simulink model "hexa_control"  (R2021a)
settings: Solver=VariableStepAuto  StartTime=0.0  StopTime=inf  RelTol=1e-3
StartFcn:
  | mikro.start('-a');
StopFcn:
  | mikro.stop();
values from neighbouring files (symbols this model uses):
  basic_time_step = 0.005    [Initialization.m]
  F = [F1; F2]    [Initialization.m]
  g = 9.81    [Initialization.m]
  J = diag([82973.961,81490.708,157588.499]*10^(-6))    [Initialization.m]
  K_p = K_p_scalar*eye(3)    [Initialization.m]
  K_R = K_R_scalar*eye(3)    [Initialization.m]
  K_v = K_v_scalar*eye(3)    [Initialization.m]
  K_w = K_w_scalar*eye(3)    [Initialization.m]
  m = 0.395 + 1.870    (= 2.265)    [Initialization.m]
  motion_capture_rate = 0.01    [Initialization.m]
undefined symbols (not defined in the file or in its folder): DiscIntNeverNeededParam, init
libraries: genomix x5, simulink x4, sharedTrackingLibrary x1
PauseFcn:
  | mikro.stop();
settings Model: Creator=nicola  LastModifiedBy=nicola

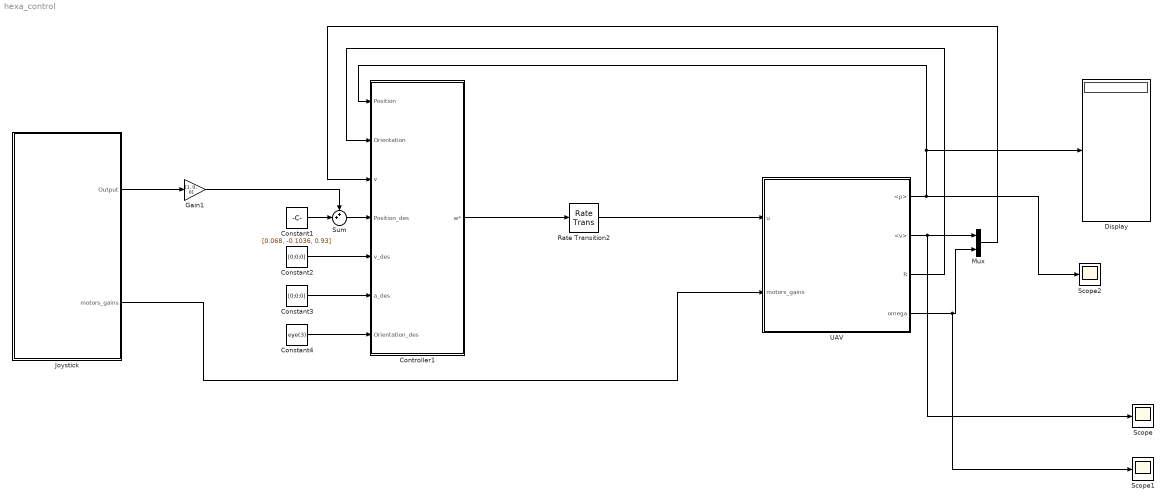
== system hexa_control ==
  Constant1 : Constant  Value=[0.068, -0.1036, 0.93]
  Constant2 : Constant  Value=[0;0;0]
  Constant3 : Constant  Value=[0;0;0]
  Constant4 : Constant  Value=eye(3)
  Controller1 : Subsystem
  Display : Display
  Gain1 : Gain  Gain=[1, 0, 0]
  Joystick : Subsystem
  Mux : Mux  Inputs=2
  Rate Transition2 : RateTransition  Integrity=off
  Scope : Scope
  Scope1 : Scope
  Scope2 : Scope
  Sum : Sum  Inputs=++|
  UAV : Subsystem
  wires:
  Controller1/1("w* ") -> Rate Transition2/1
  Constant3/1 -> Controller1/6(a_des)
  Constant1/1 -> Sum/2
  Gain1/1 -> Sum/1
  Constant2/1 -> Controller1/5(v_des)
  Sum/1 -> Controller1/4(Position_des)
  UAV/1(<p>) -> Scope2/1, Display/1, Controller1/1(Position)
  Constant4/1 -> Controller1/7(Orientation_des)
  UAV/3(R) -> Controller1/2(Orientation)
  Rate Transition2/1 -> UAV/1(u)
  UAV/2(<v>) -> Scope/1, Mux/1
  UAV/4(omega) -> Scope1/1, Mux/2
  Mux/1 -> Controller1/3(v)
  Joystick/1(Output) -> Gain1/1
  Joystick/2(motors_gains) -> UAV/2(motors_gains)

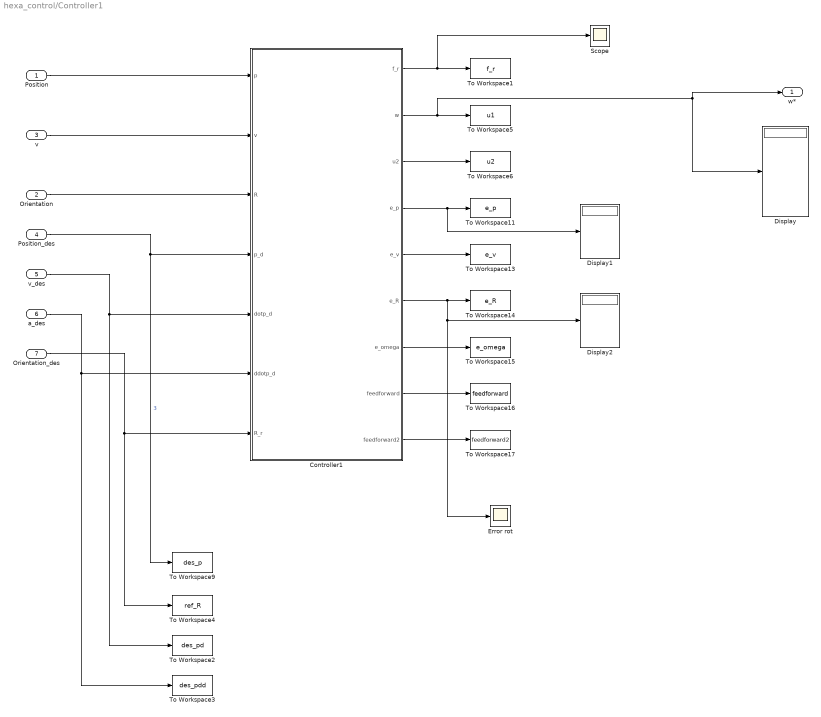
== system hexa_control/Controller1 ==
  Position : Inport
  Orientation : Inport  Port=2
  v : Inport  Port=3
  Position_des : Inport  Port=4
  v_des : Inport  Port=5
  a_des : Inport  Port=6
  Orientation_des : Inport  Port=7
  Controller1 : MATLAB Function  TreatAsAtomicUnit=on
  Display : Display
  Display1 : Display
  Display2 : Display
  Error rot : Scope
  Scope : Scope
  To Workspace1 : ToWorkspace  VariableName=f_r  SaveFormat=Timeseries  SampleTime=-1
  To Workspace11 : ToWorkspace  VariableName=e_p  SaveFormat=Timeseries  SampleTime=-1
  To Workspace13 : ToWorkspace  VariableName=e_v  SaveFormat=Timeseries  SampleTime=-1
  To Workspace14 : ToWorkspace  VariableName=e_R  SaveFormat=Timeseries  SampleTime=-1
  To Workspace15 : ToWorkspace  VariableName=e_omega  SaveFormat=Timeseries  SampleTime=-1
  To Workspace16 : ToWorkspace  VariableName=feedforward  SaveFormat=Timeseries  SampleTime=-1
  To Workspace17 : ToWorkspace  VariableName=feedforward2  SaveFormat=Timeseries  SampleTime=-1
  To Workspace2 : ToWorkspace  VariableName=des_pd  SaveFormat=Timeseries  SampleTime=-1
  To Workspace3 : ToWorkspace  VariableName=des_pdd  SaveFormat=Timeseries  SampleTime=-1
  To Workspace4 : ToWorkspace  VariableName=ref_R  SaveFormat=Timeseries  SampleTime=-1
  To Workspace5 : ToWorkspace  VariableName=u1  SaveFormat=Timeseries  SampleTime=-1
  To Workspace6 : ToWorkspace  VariableName=u2  SaveFormat=Timeseries  SampleTime=-1
  To Workspace9 : ToWorkspace  VariableName=des_p  SaveFormat=Timeseries  SampleTime=-1
  "w* " : Outport
  wires:
  Position/1 -> Controller1/1(p)
  v/1 -> Controller1/2(v)
  Orientation_des/1 -> To Workspace4/1, Controller1/7(R_r)
  Orientation/1 -> Controller1/3(R)
  Position_des/1 -> Controller1/4(p_d), To Workspace9/1  "3"
  v_des/1 -> Controller1/5(dotp_d), To Workspace2/1
  a_des/1 -> Controller1/6(ddotp_d), To Workspace3/1
  Controller1/4(e_p) -> Display1/1, To Workspace11/1
  Controller1/5(e_v) -> To Workspace13/1
  Controller1/7(e_omega) -> To Workspace15/1
  Controller1/3(u2) -> To Workspace6/1
  Controller1/2(w) -> Display/1, "w* "/1, To Workspace5/1
  Controller1/6(e_R) -> Error rot/1, Display2/1, To Workspace14/1
  Controller1/8(feedforward) -> To Workspace16/1
  Controller1/9(feedforward2) -> To Workspace17/1
  Controller1/1(f_r) -> Scope/1, To Workspace1/1

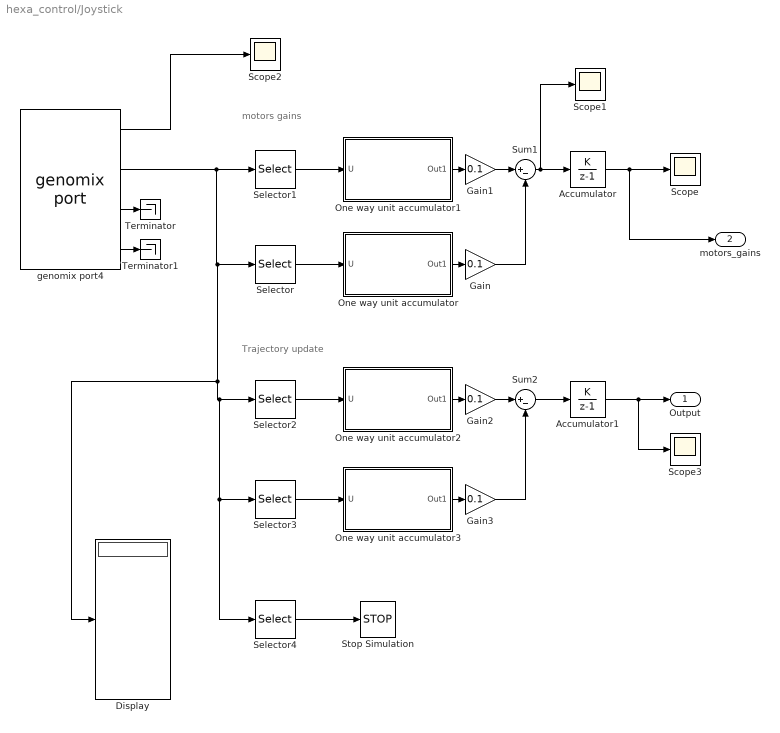
== system hexa_control/Joystick ==
  note: Trajectory update
  note: motors gains
  Accumulator : DiscreteIntegrator  IntegratorMethod=Accumulation: Forward Euler  gainval=1  SampleTime=-1  LimitOutput=on  UpperSaturationLimit=1  LowerSaturationLimit=0  ICPrevOutput=DiscIntNeverNeededParam  ICPrevScaledInput=DiscIntNeverNeededParam
  Accumulator1 : DiscreteIntegrator  IntegratorMethod=Accumulation: Forward Euler  gainval=1  SampleTime=-1  LimitOutput=on  UpperSaturationLimit=1  LowerSaturationLimit=-1  ICPrevOutput=DiscIntNeverNeededParam  ICPrevScaledInput=DiscIntNeverNeededParam
  Display : Display
  Gain{,1..3} (4 alike) : Gain  Gain=0.1
  One way unit accumulator : Subsystem
  One way unit accumulator1 : Subsystem
  One way unit accumulator2 : Subsystem
  One way unit accumulator3 : Subsystem
  Scope{,1..3} (4 alike) : Scope
  Selector : Selector  InputPortWidth=16  IndexOptions=Index vector (dialog)  Indices=[1]  OutputSizes=1
  Selector1 : Selector  InputPortWidth=16  IndexOptions=Index vector (dialog)  Indices=[2]  OutputSizes=1
  Selector2 : Selector  InputPortWidth=16  IndexOptions=Index vector (dialog)  Indices=[4]  OutputSizes=1
  Selector3 : Selector  InputPortWidth=16  IndexOptions=Index vector (dialog)  Indices=[3]  OutputSizes=1
  Selector4 : Selector  InputPortWidth=16  IndexOptions=Index vector (dialog)  Indices=[6]  OutputSizes=1
  Stop Simulation : Stop
  Sum1 : Sum  Inputs=|+-
  Sum2 : Sum  Inputs=|+-
  Terminator : Terminator
  Terminator1 : Terminator
  genomix port4 : genomix/genomix port  host=localhost  component=joystick  port=device  subport=Logitech  sigtype=value  timetype=periodic  period=basic_time_step  siglist="[{\"name\":\"device.axes\",\"type\":\"value\",\"size\":16},{\"name\":\"device.buttons\",\"type\":\"value\",\"size\":16}]"
      settings: AttributesFormatString=joystick/device  SourceProductName=genomix
  Output : Outport
  motors_gains : Outport  Port=2
  wires:
  One way unit accumulator/1(Out1) -> Gain/1
  Selector1/1 -> One way unit accumulator1/1(U)
  genomix port4/3 -> Terminator/1
  genomix port4/1 -> Scope2/1
  One way unit accumulator1/1(Out1) -> Gain1/1
  Selector/1 -> One way unit accumulator/1(U)
  genomix port4/4 -> Terminator1/1
  genomix port4/2 -> Display/1, Selector4/1, Selector3/1, Selector2/1, Selector/1, Selector1/1
  Sum1/1 -> Scope1/1, Accumulator/1
  Accumulator/1 -> motors_gains/1, Scope/1
  Gain/1 -> Sum1/2
  Gain1/1 -> Sum1/1
  Selector2/1 -> One way unit accumulator2/1(U)
  One way unit accumulator2/1(Out1) -> Gain2/1
  Selector3/1 -> One way unit accumulator3/1(U)
  One way unit accumulator3/1(Out1) -> Gain3/1
  Gain2/1 -> Sum2/1
  Gain3/1 -> Sum2/2
  Sum2/1 -> Accumulator1/1
  Accumulator1/1 -> Output/1, Scope3/1
  Selector4/1 -> Stop Simulation/1

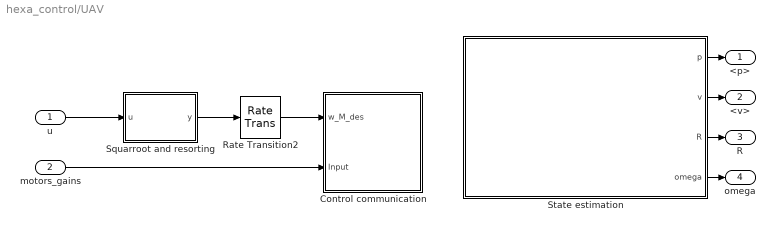
== system hexa_control/UAV ==
  u : Inport
  motors_gains : Inport  Port=2
  Control communication : Subsystem
  Rate Transition2 : RateTransition  Deterministic=off  InitialCondition=[0 0 0 0 0 0]
  Squarroot and resorting : MATLAB Function  TreatAsAtomicUnit=on
  State estimation : Subsystem
  <p> : Outport
  <v> : Outport  Port=2
  R : Outport  Port=3
  omega : Outport  Port=4
  wires:
  State estimation/1(p) -> <p>/1
  Squarroot and resorting/1(y) -> Rate Transition2/1
  State estimation/3(R) -> R/1
  State estimation/2(v) -> <v>/1
  Rate Transition2/1 -> Control communication/1(w_M_des)
  State estimation/4(omega) -> omega/1
  u/1 -> Squarroot and resorting/1(u)
  motors_gains/1 -> Control communication/2(Input)

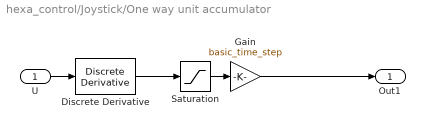
== system hexa_control/Joystick/One way unit accumulator ==
  U : Inport
  Discrete Derivative : simulink/Discrete/Discrete Derivative  gainval=1.0  ICPrevScaledInput=0.0  OutMin=[]  OutMax=[]  OutDataType=fixdt(1, 16)  OutScaling=2^-10  DoSatur=off
  Gain : Gain  Gain=basic_time_step
  Saturation : Saturate  UpperLimit=inf  LowerLimit=0
  Out1 : Outport
  wires:
  U/1 -> Discrete Derivative/1
  Gain/1 -> Out1/1
  Saturation/1 -> Gain/1
  Discrete Derivative/1 -> Saturation/1

== system hexa_control/Joystick/One way unit accumulator1 ==
  U : Inport
  Discrete Derivative : simulink/Discrete/Discrete Derivative  gainval=1.0  ICPrevScaledInput=0.0  OutMin=[]  OutMax=[]  OutDataType=fixdt(1, 16)  OutScaling=2^-10  DoSatur=off
  Gain : Gain  Gain=basic_time_step
  Saturation : Saturate  UpperLimit=inf  LowerLimit=0
  Out1 : Outport
  wires:
  Discrete Derivative/1 -> Saturation/1
  Saturation/1 -> Gain/1
  Gain/1 -> Out1/1
  U/1 -> Discrete Derivative/1

== system hexa_control/Joystick/One way unit accumulator2 ==
  U : Inport
  Discrete Derivative : simulink/Discrete/Discrete Derivative  gainval=1.0  ICPrevScaledInput=0.0  OutMin=[]  OutMax=[]  OutDataType=fixdt(1, 16)  OutScaling=2^-10  DoSatur=off
  Gain : Gain  Gain=basic_time_step
  Saturation : Saturate  UpperLimit=inf  LowerLimit=0
  Out1 : Outport
  wires:
  Discrete Derivative/1 -> Saturation/1
  Saturation/1 -> Gain/1
  Gain/1 -> Out1/1
  U/1 -> Discrete Derivative/1

== system hexa_control/Joystick/One way unit accumulator3 ==
  U : Inport
  Discrete Derivative : simulink/Discrete/Discrete Derivative  gainval=1.0  ICPrevScaledInput=0.0  OutMin=[]  OutMax=[]  OutDataType=fixdt(1, 16)  OutScaling=2^-10  DoSatur=off
  Gain : Gain  Gain=basic_time_step
  Saturation : Saturate  UpperLimit=inf  LowerLimit=0
  Out1 : Outport
  wires:
  Discrete Derivative/1 -> Saturation/1
  Saturation/1 -> Gain/1
  Gain/1 -> Out1/1
  U/1 -> Discrete Derivative/1

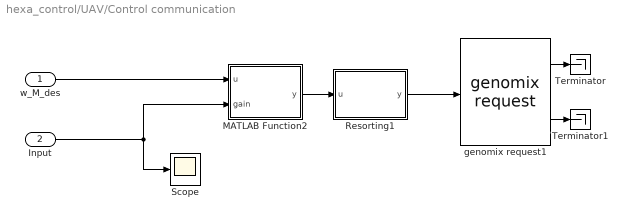
== system hexa_control/UAV/Control communication ==
  w_M_des : Inport
  Input : Inport  Port=2
  MATLAB Function2 : MATLAB Function  TreatAsAtomicUnit=on
  Resorting1 : MATLAB Function  TreatAsAtomicUnit=on
  Scope : Scope
  Terminator : Terminator
  Terminator1 : Terminator
  genomix request1 : genomix/genomix request  host=localhost  path=/opt/openrobots/lib/genom/pocolibs/plugins/  component=rotorcraft  port=set_velocity  sigtype=value  timetype=periodic  period=basic_time_step  siglist="[{\"name\":\"desired\",\"type\":\"value\",\"size\":8}]"
      settings: AttributesFormatString=rotorcraft/set_velocity  SourceProductName=genomix
  wires:
  genomix request1/2 -> Terminator1/1
  Resorting1/1(y) -> genomix request1/1
  genomix request1/1 -> Terminator/1
  w_M_des/1 -> MATLAB Function2/1(u)
  MATLAB Function2/1(y) -> Resorting1/1(u)
  Input/1 -> Scope/1, MATLAB Function2/2(gain)

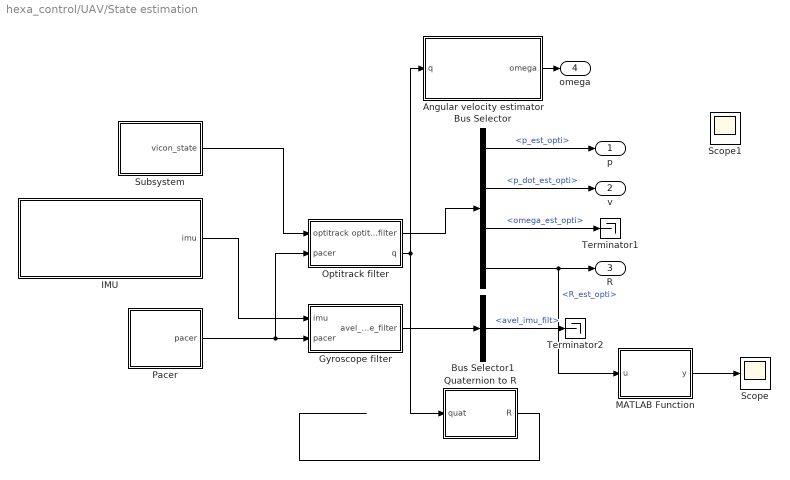
== system hexa_control/UAV/State estimation ==
  Angular velocity estimator : Subsystem
  Bus Selector : BusSelector  OutputSignals=linear.p_est_opti,linear.p_dot_est_opti,angular.omega_est_opti,angular.R_est_opti
  Bus Selector1 : BusSelector  OutputSignals=avel_imu_filt
  Gyroscope filter : Subsystem
  IMU : Subsystem
  MATLAB Function : MATLAB Function  TreatAsAtomicUnit=on
  Optitrack filter : Subsystem
  Pacer : Subsystem
  Quaternion to R : MATLAB Function  SystemSampleTime=motion_capture_rate
  Scope : Scope
  Scope1 : Scope
  Subsystem : Subsystem
  Terminator1 : Terminator
  Terminator2 : Terminator
  p : Outport
  v : Outport  Port=2
  R : Outport  Port=3
  omega : Outport  Port=4
  wires:
  Subsystem/1(vicon_state) -> Optitrack filter/1(optitrack)
  Optitrack filter/1(optitrack_filter) -> Bus Selector/1
  Optitrack filter/2(q) -> Quaternion to R/1(quat), Angular velocity estimator/1(q)
  Bus Selector1/1 -> Terminator2/1  "<avel_imu_filt>"
  Gyroscope filter/1(avel_gyroscope_filter) -> Bus Selector1/1
  IMU/1(imu) -> Gyroscope filter/1(imu)
  Pacer/1(pacer) -> Optitrack filter/2(pacer), Gyroscope filter/2(pacer)
  Angular velocity estimator/1(omega) -> omega/1
  Quaternion to R/1(R) -> ?
  MATLAB Function/1(y) -> Scope/1
  Bus Selector/1 -> p/1  "<p_est_opti>"
  Bus Selector/2 -> v/1  "<p_dot_est_opti>"
  Bus Selector/3 -> Terminator1/1  "<omega_est_opti>"
  Bus Selector/4 -> MATLAB Function/1(u), R/1  "<R_est_opti>"

== system hexa_control/UAV/State estimation/Angular velocity estimator ==
  q : Inport
  Extended Kalman Filter : sharedTrackingLibrary/Extended Kalman Filter  StateTransitionFcn=ekf_model  HasStateTransitionJacobianFcn=off  HasAdditiveProcessNoise=Additive  ProcessNoise=0.01*diag([0, 0, 0, 0, 1, 1, 1])  HasTimeVaryingProcessNoise=off  HasStateTransitionFcnExtraArgument=0  InitialState=[1, 0, 0, 0, 0, 0, 0]'  InitialStateCovariance=1  MeasurementFcn1=output_quat  HasMeasurementJacobianFcn1=off  HasMeasurementEnablePort1=off  HasAdditiveMeasurementNoise1=Additive  MeasurementNoise1=eye(4)*0.0001  HasTimeVaryingMeasurementNoise1=off  HasMeasurementFcnExtraArgument1=0  MeasurementFcn2=myMeasurementFcn  HasMeasurementJacobianFcn2=off  HasMeasurementEnablePort2=off  HasAdditiveMeasurementNoise2=Additive  MeasurementNoise2=1  HasTimeVaryingMeasurementNoise2=off  HasMeasurementFcnExtraArgument2=0  MeasurementFcn3=myMeasurementFcn  HasMeasurementJacobianFcn3=off  HasMeasurementEnablePort3=off  HasAdditiveMeasurementNoise3=Additive  MeasurementNoise3=1  HasTimeVaryingMeasurementNoise3=off  HasMeasurementFcnExtraArgument3=0  MeasurementFcn4=myMeasurementFcn  HasMeasurementJacobianFcn4=off  HasMeasurementEnablePort4=off  HasAdditiveMeasurementNoise4=Additive  MeasurementNoise4=1  HasTimeVaryingMeasurementNoise4=off  HasMeasurementFcnExtraArgument4=0  MeasurementFcn5=myMeasurementFcn  HasMeasurementJacobianFcn5=off  HasMeasurementEnablePort5=off  HasAdditiveMeasurementNoise5=Additive  MeasurementNoise5=1  HasTimeVaryingMeasurementNoise5=off  HasMeasurementFcnExtraArgument5=0  EnableMultirate=off  StateTransitionFcnSampleTime=1  MeasurementFcn1SampleTime=1  MeasurementFcn2SampleTime=1  MeasurementFcn3SampleTime=1  MeasurementFcn4SampleTime=1  MeasurementFcn5SampleTime=1  UseCurrentEstimator=on  OutputStateCovariance=off  DataType=double  SampleTime=0.01  NumberOfMeasurements=1
      settings: SourceProductBaseCode=CT,DR,TF,ID,LP,NV,AR,RO,RR,UV,VE
  Selector : Selector  InputPortWidth=7  IndexOptions=Index vector (dialog)  Indices=[5 6 7]  OutputSizes=1
  Zero-Order Hold : ZeroOrderHold  SampleTime=0.01
  omega : Outport
  wires:
  Extended Kalman Filter/1 -> Selector/1
  Zero-Order Hold/1 -> Extended Kalman Filter/1
  Selector/1 -> omega/1
  q/1 -> Zero-Order Hold/1

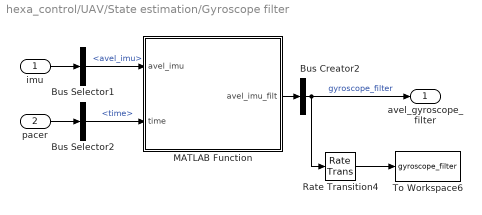
== system hexa_control/UAV/State estimation/Gyroscope filter ==
  imu : Inport
  pacer : Inport  Port=2
  Bus Creator2 : BusCreator  Inputs=1
  Bus Selector1 : BusSelector  OutputSignals=avel_imu
  Bus Selector2 : BusSelector  OutputSignals=time
  MATLAB Function : MATLAB Function  TreatAsAtomicUnit=on
  Rate Transition4 : RateTransition  InitialCondition=-1  OutPortSampleTime=init.log_time_step
  To Workspace6 : ToWorkspace  VariableName=gyroscope_filter  SaveFormat=Timeseries  SampleTime=init.log_time_step
  avel_gyroscope_filter : Outport  VectorParamsAs1DForOutWhenUnconnected=off
  wires:
  imu/1 -> Bus Selector1/1
  MATLAB Function/1(avel_imu_filt) -> Bus Creator2/1
  pacer/1 -> Bus Selector2/1
  Bus Selector1/1 -> MATLAB Function/1(avel_imu)  "<avel_imu>"
  Bus Selector2/1 -> MATLAB Function/2(time)  "<time>"
  Bus Creator2/1 -> Rate Transition4/1, avel_gyroscope_filter/1  "gyroscope_filter"
  Rate Transition4/1 -> To Workspace6/1

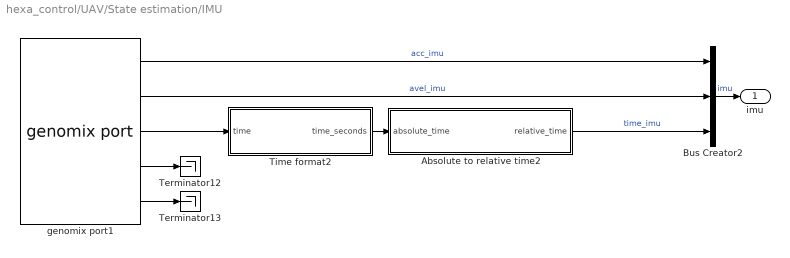
== system hexa_control/UAV/State estimation/IMU ==
  Absolute to relative time2 : MATLAB Function  TreatAsAtomicUnit=on
  Bus Creator2 : BusCreator  Inputs=3
  Terminator12 : Terminator
  Terminator13 : Terminator
  Time format2 : MATLAB Function  TreatAsAtomicUnit=on
  genomix port1 : genomix/genomix port  host=localhost  path=/opt/openrobots/lib/genom/pocolibs/plugins/  component=rotorcraft  port=imu  sigtype=value  timetype=periodic  period=init.time_step  siglist="[{\"name\":\"imu.acc\",\"type\":\"value\",\"size\":3},{\"name\":\"imu.avel\",\"type\":\"value\",\"size\":3},{\"name\":\"imu.ts\",\"type\":\"value\",\"size\":2}]"
      settings: AttributesFormatString=rotorcraft/imu  SourceProductName=genomix
  imu : Outport
  wires:
  genomix port1/1 -> Bus Creator2/1  "acc_imu"
  genomix port1/3 -> Time format2/1(time)
  genomix port1/2 -> Bus Creator2/2  "avel_imu"
  Bus Creator2/1 -> imu/1  "imu"
  Time format2/1(time_seconds) -> Absolute to relative time2/1(absolute_time)
  Absolute to relative time2/1(relative_time) -> Bus Creator2/3  "time_imu"
  genomix port1/4 -> Terminator12/1
  genomix port1/5 -> Terminator13/1

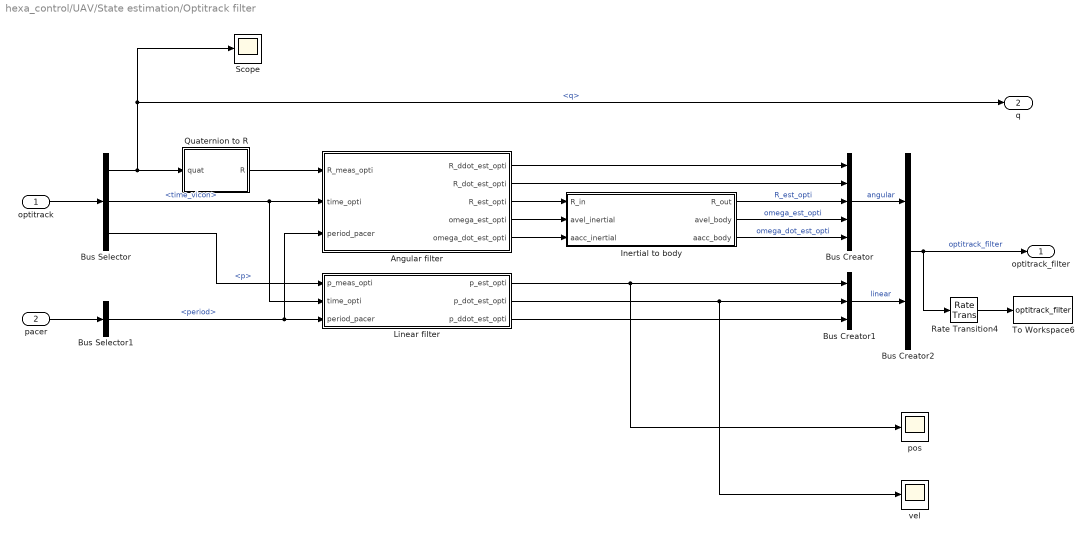
== system hexa_control/UAV/State estimation/Optitrack filter ==
  optitrack : Inport
  pacer : Inport  Port=2
  Angular filter : MATLAB Function  TreatAsAtomicUnit=on
  Bus Creator : BusCreator  Inputs=5
  Bus Creator1 : BusCreator  Inputs=3
  Bus Creator2 : BusCreator  Inputs=2
  Bus Selector : BusSelector  OutputSignals=q,time_vicon,p
  Bus Selector1 : BusSelector  OutputSignals=period
  Inertial to body : MATLAB Function  SystemSampleTime=motion_capture_rate
  Linear filter : MATLAB Function  TreatAsAtomicUnit=on
  Quaternion to R : MATLAB Function  SystemSampleTime=motion_capture_rate
  Rate Transition4 : RateTransition  InitialCondition=-1  OutPortSampleTime=init.log_time_step
  Scope : Scope
  To Workspace6 : ToWorkspace  VariableName=optitrack_filter  SaveFormat=Timeseries  SampleTime=init.log_time_step
  pos : Scope
  vel : Scope
  optitrack_filter : Outport  VectorParamsAs1DForOutWhenUnconnected=off
  q : Outport  Port=2
  wires:
  Bus Selector/3 -> Linear filter/1(p_meas_opti)  "<p>"
  Bus Selector/1 -> q/1, Scope/1, Quaternion to R/1(quat)  "<q>"
  Bus Selector1/1 -> Linear filter/3(period_pacer), Angular filter/3(period_pacer)  "<period>"
  Bus Selector/2 -> Linear filter/2(time_opti), Angular filter/2(time_opti)  "<time_vicon>"
  Linear filter/3(p_ddot_est_opti) -> Bus Creator1/3
  Quaternion to R/1(R) -> Angular filter/1(R_meas_opti)
  pacer/1 -> Bus Selector1/1
  Linear filter/1(p_est_opti) -> pos/1, Bus Creator1/1
  optitrack/1 -> Bus Selector/1
  Linear filter/2(p_dot_est_opti) -> vel/1, Bus Creator1/2
  Bus Creator/1 -> Bus Creator2/1  "angular"
  Angular filter/3(R_est_opti) -> Inertial to body/1(R_in)
  Angular filter/4(omega_est_opti) -> Inertial to body/2(avel_inertial)
  Angular filter/5(omega_dot_est_opti) -> Inertial to body/3(aacc_inertial)
  Inertial to body/3(aacc_body) -> Bus Creator/5  "omega_dot_est_opti"
  Inertial to body/2(avel_body) -> Bus Creator/4  "omega_est_opti"
  Inertial to body/1(R_out) -> Bus Creator/3  "R_est_opti"
  Angular filter/2(R_dot_est_opti) -> Bus Creator/2
  Angular filter/1(R_ddot_est_opti) -> Bus Creator/1
  Bus Creator1/1 -> Bus Creator2/2  "linear"
  Bus Creator2/1 -> Rate Transition4/1, optitrack_filter/1  "optitrack_filter"
  Rate Transition4/1 -> To Workspace6/1

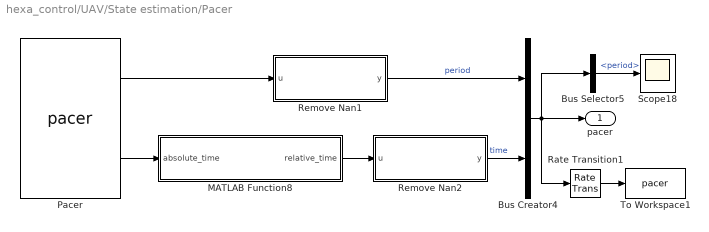
== system hexa_control/UAV/State estimation/Pacer ==
  Bus Creator4 : BusCreator  Inputs=2
  Bus Selector5 : BusSelector  OutputSignals=period
  MATLAB Function8 : MATLAB Function  TreatAsAtomicUnit=on
  Pacer : genomix/pacer  Priority=0  catchup=off
      settings: SourceProductName=genomix
  Rate Transition1 : RateTransition  InitialCondition=-1  OutPortSampleTime=init.log_time_step
  Remove Nan1 : MATLAB Function  SystemSampleTime=motion_capture_rate
  Remove Nan2 : MATLAB Function  SystemSampleTime=motion_capture_rate
  Scope18 : Scope
  To Workspace1 : ToWorkspace  VariableName=pacer  SaveFormat=Timeseries  SampleTime=init.log_time_step
  pacer : Outport
  wires:
  Pacer/1 -> Remove Nan1/1(u)
  Remove Nan1/1(y) -> Bus Creator4/1  "period"
  Pacer/2 -> MATLAB Function8/1(absolute_time)
  MATLAB Function8/1(relative_time) -> Remove Nan2/1(u)
  Bus Selector5/1 -> Scope18/1  "<period>"
  Rate Transition1/1 -> To Workspace1/1
  Bus Creator4/1 -> pacer/1, Rate Transition1/1, Bus Selector5/1
  Remove Nan2/1(y) -> Bus Creator4/2  "time"

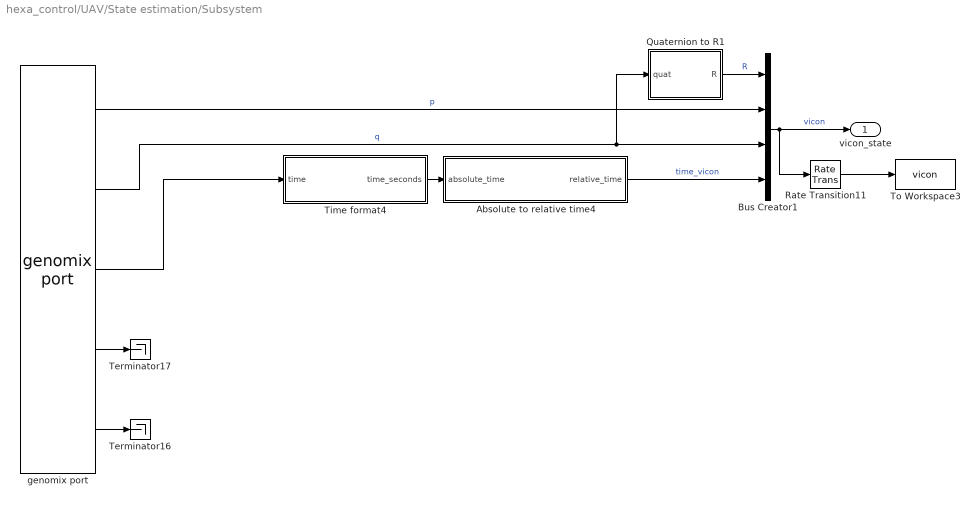
== system hexa_control/UAV/State estimation/Subsystem ==
  Absolute to relative time4 : MATLAB Function  TreatAsAtomicUnit=on
  Bus Creator1 : BusCreator  Inputs=4
  Quaternion to R1 : MATLAB Function  SystemSampleTime=motion_capture_rate
  Rate Transition11 : RateTransition  InitialCondition=-1  OutPortSampleTime=init.log_time_step
  Terminator16 : Terminator
  Terminator17 : Terminator
  Time format4 : MATLAB Function  TreatAsAtomicUnit=on
  To Workspace3 : ToWorkspace  VariableName=vicon  SaveFormat=Timeseries  SampleTime=init.log_time_step
  genomix port : genomix/genomix port  host=localhost  path=/opt/openrobots/lib/genom/pocolibs/plugins/  component=vicon  port=bodies  subport=Hexa  sigtype=value  timetype=periodic  period=basic_time_step  siglist="[{\"name\":\"bodies.pos\",\"type\":\"value\",\"size\":3},{\"name\":\"bodies.att\",\"type\":\"value\",\"size\":4},{\"name\":\"bodies.ts\",\"type\":\"value\",\"size\":2}]"
      settings: AttributesFormatString=vicon/bodies  SourceProductName=genomix
  vicon_state : Outport  VectorParamsAs1DForOutWhenUnconnected=off
  wires:
  Absolute to relative time4/1(relative_time) -> Bus Creator1/4  "time_vicon"
  Quaternion to R1/1(R) -> Bus Creator1/1  "R"
  genomix port/2 -> Quaternion to R1/1(quat), Bus Creator1/3  "q"
  Bus Creator1/1 -> Rate Transition11/1, vicon_state/1  "vicon"
  Time format4/1(time_seconds) -> Absolute to relative time4/1(absolute_time)
  Rate Transition11/1 -> To Workspace3/1
  genomix port/3 -> Time format4/1(time)
  genomix port/1 -> Bus Creator1/2  "p"
  genomix port/4 -> Terminator17/1
  genomix port/5 -> Terminator16/1

== matlab function hexa_control/UAV/Control communication/MATLAB Function2 ==
  data: u input; y output; gain input
function y = fcn(u,gain)
%#codegen

y=gain*u;

== matlab function hexa_control/UAV/State estimation/Subsystem/Time format4 ==
  data: time input; time_seconds output
function time_seconds = time_format( time )

time_seconds = time(1) + time(2)*1e-9;

== matlab function hexa_control/UAV/State estimation/Subsystem/Absolute to relative time4 ==
  data: absolute_time input; relative_time output
function relative_time = absolute_to_relative_time( absolute_time )

persistent initial_time;
if( isempty(initial_time) )
    initial_time = absolute_time;
end

relative_time = absolute_time - initial_time;

end

== matlab function hexa_control/UAV/State estimation/IMU/Absolute to relative time2 ==
  data: absolute_time input; relative_time output
function relative_time = absolute_to_relative_time( absolute_time )

persistent initial_time;
if( isempty(initial_time) )
    initial_time = absolute_time;
end

relative_time = absolute_time - initial_time;

end

== matlab function hexa_control/UAV/State estimation/Quaternion to R ==
  data: quat input double size=[4,1]; R output double size=[3,3]
function R = quatToR( quat )
%qv = quat(2:4,1);
%qs = quat(1,1);
%q = [qv; qs];

R = quat2rotm( quat' )';

== matlab function hexa_control/UAV/State estimation/Optitrack filter/Angular filter ==
  data: R_ddot_est_opti output double size=[3,3]; R_dot_est_opti output double size=[3,3]; R_est_opti output double size=[3,3]; R_meas_opti input double size=[3,3]; time_opti input double size=1; omega_est_opti output double size=[3,1]; omega_dot_est_opti output double size=[3,1]; period_pacer input double size=1
% % % function [p_est_opti,p_dot_est_opti,p_ddot_est_opti] = fcn(p_meas_opti,time_opti)
function [R_ddot_est_opti,R_dot_est_opti,R_est_opti,omega_est_opti,omega_dot_est_opti] = fcn(R_meas_opti,time_opti,period_pacer)

% coder.extrinsic('quadprog'); 
% n = 4;
n = 9;

persistent counter;
if(isempty(counter))
    counter = 0;
end

persistent a;
if(isempty(a))
    a = zeros(3,1);
end
persistent b;
if(isempty(b))
    b = zeros(3,1);
end
persistent c;
if(isempty(c))
    c = zeros(3,1);
end

persistent old_omega;
if(isempty(old_omega))
    old_omega = zeros(3,1);
end
persistent old_omega_dot;
if(isempty(old_omega_dot))
    old_omega_dot = zeros(3,1);
end
persistent old_buffer;
if(isempty(old_buffer))
    old_buffer = zeros(n,10);
end

if time_opti~=old_buffer(1,1) % if I have a new measurement
    buffer = [time_opti,reshape(R_meas_opti,1,9);old_buffer(1:n-1,:)];
    %%%%%%%%%%%%%%%%%%%%%%%%%%%%%%%%%%%%%%%%%%%%%%%%%%%%%%%%%%%%%%%%%%%%%%%
    Y = reshape((flipud(buffer(:,2:end)))',9*n,1);
    A = zeros(9*n,27);
    for i = 1:n
        A_i = [buffer(n-i+1,1)^2*eye(9),buffer(n-i+1,1)*eye(9),eye(9)];
        A(9*i-8:9*i,:) = A_i;
    end
% %     R = eye(3*n);
% %     H = 2*A'*R*A;
% %     f_transp = -2*Y'*R*A;
% %     x = zeros(9,1); % very important to initialize the values, which otherwise would be an mxArray
% %     x = quadprog(H,f_transp);
    x = A\Y;
    a = x(1:9);
    b = x(10:18);
    c = x(19:27);
    %%%%%%%%%%%%%%%%%%%%%%%%%%%%%%%%%%%%%%%%%%%%%%%%%%%%%%%%%%%%%%%%%%%%%%%
    flag = all(buffer(1:end-1,1)); % if the buffer has not be completely filled, I set the estimation to zeros(3,1)
    if ~flag
        R_est_opti = R_meas_opti;
        R_dot_est_opti = zeros(3,3);
        R_ddot_est_opti = zeros(3,3);
    else
        R_est_opti = reshape(a*time_opti^2+b*time_opti+c,3,3);
        %%%%%%%% Othonormalizing R_est_opti %%%%%%%%
        
        %%%%%%%%%%%%%%%%%%%%%%%%%%%%%%%%%%%%%%%%%%%%
        R_dot_est_opti = reshape(2*a*time_opti+b,3,3);
        R_ddot_est_opti = reshape(2*a,3,3);
    end
    
    S_omega = R_est_opti'*R_dot_est_opti;
    S_omega = 0.5 * (S_omega - S_omega'); % I force the matrix to be skew-symmetric
    omega_est_opti = [-S_omega(2,3); S_omega(1,3); -S_omega(1,2)];
    
    S_alpha = R_est_opti'*(R_ddot_est_opti-R_dot_est_opti*S_omega);
    S_alpha = 0.5 * (S_alpha - S_alpha'); % I force the matrix to be skew-symmetric
    omega_dot_est_opti = [-S_alpha(2,3); S_alpha(1,3); -S_alpha(1,2)];
    
    % update
    old_buffer = buffer;

    old_omega = omega_est_opti;
    old_omega_dot = omega_dot_est_opti;
    counter = 0; % reset the counter
else % else if I don't have a new measument
    buffer = [time_opti,reshape(R_meas_opti,1,9);old_buffer(1:n-1,:)];
    flag = all(buffer(1:end-1,1)); % if the buffer has not be completely filled
    if ~flag
        R_est_opti = R_meas_opti;
        R_dot_est_opti = zeros(3,3);
        R_ddot_est_opti = zeros(3,3);
        omega_est_opti = old_omega;
        omega_dot_est_opti = old_omega_dot;
    else
        counter = counter+period_pacer;
        R_est_opti = reshape(a*(time_opti+counter)^2+b*(time_opti+counter)+c,3,3);
        %%%%%%%% Othonormalizing R_est_opti %%%%%%%%
        
        %%%%%%%%%%%%%%%%%%%%%%%%%%%%%%%%%%%%%%%%%%%%
        R_dot_est_opti = reshape(2*a*(time_opti+counter)+b,3,3);
        R_ddot_est_opti = reshape(2*a,3,3);
        
        S_omega = R_est_opti'*R_dot_est_opti;
        S_omega = 0.5 * (S_omega - S_omega'); % I force the matrix to be skew-symmetric
        omega_est_opti = [-S_omega(2,3); S_omega(1,3); -S_omega(1,2)];

        S_alpha = R_est_opti'*(R_ddot_est_opti-R_dot_est_opti*S_omega);
        S_alpha = 0.5 * (S_alpha - S_alpha'); % I force the matrix to be skew-symmetric
        omega_dot_est_opti = [-S_alpha(2,3); S_alpha(1,3); -S_alpha(1,2)];
    end
%     omega_est_opti = old_omega;
%     omega_dot_est_opti = old_omega_dot;

end

== matlab function hexa_control/UAV/State estimation/Optitrack filter/Quaternion to R ==
  data: quat input double size=[4,1]; R output double size=[3,3]
function R = quatToR( quat )
%qv = quat(2:4,1);
%qs = quat(1,1);
%q = [qv; qs];

R = quat2rotm( quat' )';

== matlab function hexa_control/UAV/State estimation/MATLAB Function ==
  data: u input; y output
function y = fcn(u)

y = rotm2eul (u,'XYZ') / (pi) * 180;

== matlab function hexa_control/UAV/Control communication/Resorting1 ==
  data: u input; y output
function y = fcn(u)
%#codegen

y = [u(1) u(2) u(3) u(4) u(5) u(6) 0 0]';

if isnan(sum(y(1:6)))
    y=[0 0 0 0 0 0 0 0]';
end

== matlab function hexa_control/UAV/State estimation/Optitrack filter/Inertial to body ==
  data: R_out output double size=[3,3]; R_in input double size=[3,3]; avel_inertial input double size=[3,1]; avel_body output double size=[3,1]; aacc_inertial input; aacc_body output
function [R_out, avel_body, aacc_body] = inertial_to_body( R_in, avel_inertial, aacc_inertial)
R_out = R_in;

avel_body = R_in * avel_inertial;
aacc_body = R_in * aacc_inertial;

== matlab function hexa_control/UAV/State estimation/Subsystem/Quaternion to R1 ==
  data: quat input double size=[4,1]; R output double size=[3,3]
function R = quatToR( quat )
%qv = quat(2:4,1);
%qs = quat(1,1);
%q = [qv; qs];

R = quat2rotm( quat' )';

== matlab function hexa_control/UAV/State estimation/Optitrack filter/Linear filter ==
  data: p_est_opti output double size=[3,1]; p_meas_opti input double size=[3,1]; time_opti input double size=1; p_dot_est_opti output double size=[3,1]; p_ddot_est_opti output double size=[3,1]; period_pacer input double size=1
function [p_est_opti,p_dot_est_opti,p_ddot_est_opti] = fcn(p_meas_opti,time_opti,period_pacer)
% % % function [p_dot_est_opti,p_ddot_est_opti] = fcn(p_meas_opti,time_opti)

% coder.extrinsic('quadprog'); 
% n = 4;
n = 9;

persistent counter;
if(isempty(counter))
    counter = 0;
end

persistent a;
if(isempty(a))
    a = zeros(3,1);
end
persistent b;
if(isempty(b))
    b = zeros(3,1);
end
persistent c;
if(isempty(c))
    c = zeros(3,1);
end

persistent old_p_dot;
if(isempty(old_p_dot))
    old_p_dot = zeros(3,1);
end
persistent old_p_ddot;
if(isempty(old_p_ddot))
    old_p_ddot = zeros(3,1);
end
persistent old_buffer;
if(isempty(old_buffer))
    old_buffer = zeros(n,4);
end

if time_opti~=old_buffer(1,1) % if I have a new measurement
    buffer = [time_opti,p_meas_opti';old_buffer(1:n-1,:)];
    %%%%%%%%%%%%%%%%%%%%%%%%%%%%%%%%%%%%%%%%%%%%%%%%%%%%%%%%%%%%%%%%%%%%%%%
    Y = reshape((flipud(buffer(:,2:4)))',3*n,1);
    A = zeros(3*n,9);
    for i = 1:n
        A_i = [buffer(n-i+1,1)^2*eye(3),buffer(n-i+1,1)*eye(3),eye(3)];
        A(3*i-2:3*i,:) = A_i;
    end
%     R = eye(3*n);
%     H = 2*A'*R*A;
%     f_transp = -2*Y'*R*A;
%     x = zeros(9,1); % very important to initialize the values, which otherwise would be an mxArray
%     x = quadprog(H,f_transp);
    x = A\Y;
    a = x(1:3);
    b = x(4:6);
    c = x(7:9);
    %%%%%%%%%%%%%%%%%%%%%%%%%%%%%%%%%%%%%%%%%%%%%%%%%%%%%%%%%%%%%%%%%%%%%%%
    flag = all(buffer(1:end-1,1)); % if the buffer has not be completely filled, I set the estimation to zeros(3,1)
    if ~flag
        p_est_opti = p_meas_opti;
        p_dot_est_opti = zeros(3,1);
        p_ddot_est_opti = zeros(3,1);
    else
        p_est_opti = a*time_opti^2+b*time_opti+c;
        p_dot_est_opti = 2*a*time_opti+b;
        p_ddot_est_opti = 2*a;
    end
    % update
    old_buffer = buffer;

    old_p_dot = p_dot_est_opti;
    old_p_ddot = p_ddot_est_opti;
    counter = 0;
else % else if I don't have a new measument
    buffer = [time_opti,p_meas_opti';old_buffer(1:n-1,:)];
    flag = all(buffer(1:end-1,1)); % if the buffer has not be completely filled
    if ~flag
        p_est_opti = p_meas_opti;
        p_dot_est_opti = zeros(3,1);
        p_ddot_est_opti = zeros(3,1);
    else
        counter = counter+period_pacer;
        p_est_opti = a*(time_opti+counter)^2+b*(time_opti+counter)+c;
        p_dot_est_opti = 2*a*(time_opti+counter)+b;
        p_ddot_est_opti = old_p_ddot;
    end
%     p_dot_est_opti = old_p_dot;
%     p_ddot_est_opti = old_p_ddot;
end

== matlab function hexa_control/UAV/State estimation/Gyroscope filter/MATLAB Function ==
  settings: updateMethod=DISCRETE  sampleTime=1/1000
  data: avel_imu input double size=[3,1]; avel_imu_filt output double size=[3,1]; time input double size=1
function avel_imu_filt = fcn(avel_imu, time)
%%
linear = 1;
badfreq_vec = [ 65 85 130 170];
ang_acc_th = 15;
window_regression = 4;

if linear == 1
    size_b_good = 2;
else
    size_b_good = 3;
end

size_b_bad = 2 * length(badfreq_vec); %two coefficients for each frequency
sample_num = window_regression * (size_b_bad + size_b_good);

%%
persistent counter;
if(isempty(counter))
    counter = 0;
end

persistent avel_imu_old;
if(isempty(avel_imu_old))
    avel_imu_old = zeros(3,1);
end

persistent time_window;
if(isempty(time_window))
    time_window = zeros(1, sample_num);
end

persistent avel_window;
if(isempty(avel_window))
    avel_window = zeros(3, sample_num);
end

%% Takes data
time_window = [time_window(1,2:end), time];
avel_window = [avel_window(:,2:end), avel_imu];

%%
if counter == sample_num    
    if linear == 1
        X_good = [ones(sample_num, 1) time_window'];
    else
        X_good = [ones(sample_num, 1) time_window' time_window'.^2];
    end
    X_bad = [sin(2*pi*time_window'*badfreq_vec) cos(2*pi*time_window'*badfreq_vec)];
    X = [X_bad X_good];
    
    new_b = X\avel_window';
    
    b_bad = new_b(1:size_b_bad,:);
    b_good = new_b(size_b_bad+1:end,:);
    
    disturb_reg = X_bad * b_bad;
    signal_reg = X_good * b_good;
    
    noise_out = reshape(disturb_reg(end,:),[3,1]);
    avel_imu_out = reshape(signal_reg(end,:),[3,1]);
    
    %% Low pass filter with adaptive bandwidth
    if linear == 1
        abs_acc_ang = diag([abs(b_good(2,1)), ...
                            abs(b_good(2,2)), ...
                            abs(b_good(2,3))]);
    else
        abs_acc_ang = diag([abs(b_good(2,1) + 2*b_good(3,1)*time_window(end)), ...
                            abs(b_good(2,2) + 2*b_good(3,2)*time_window(end)), ...
                            abs(b_good(2,3) + 2*b_good(3,3)*time_window(end))]);
    end
    ff = min(abs_acc_ang/ang_acc_th, 1);
    avel_imu_filt = (eye(3) - ff) * avel_imu_old  + ff * avel_imu_out;
%     avel_imu_filt(3) = avel_imu(3);
else
    noise_out = zeros(3, 1);
    avel_imu_out = zeros(3, 1);
    counter = counter + 1;
    avel_imu_filt = avel_imu;
end
avel_imu_old = avel_imu_filt;

end

== matlab function hexa_control/UAV/State estimation/Pacer/Remove Nan1 ==
  data: u input double size=1; y output double size=1
function y = period_nan_remover( u )

if isnan( u )
    y = 0;
else
    y = u;
end

== matlab function hexa_control/UAV/State estimation/Pacer/Remove Nan2 ==
  data: u input; y output
function y = time_nan_remover( u )

persistent last_useful_data_pers;
if isempty(last_useful_data_pers)
    last_useful_data_pers = u;
end

if isnan(u)
    y = last_useful_data_pers;
else
    y = u;
    last_useful_data_pers = u;
end

end

== matlab function hexa_control/UAV/State estimation/Pacer/MATLAB Function8 ==
  data: absolute_time input; relative_time output
function relative_time = absolute_to_relative_time( absolute_time )

persistent initial_time;
if( isempty(initial_time) )
    initial_time = absolute_time;
end

relative_time = absolute_time - initial_time;

end

== matlab function hexa_control/UAV/State estimation/IMU/Time format2 ==
  data: time input; time_seconds output
function time_seconds = time_format( time )

time_seconds = time(1) + time(2)*1e-9;

== matlab function hexa_control/UAV/Squarroot and resorting ==
  data: u input; y output
function y = fcn(u)
%#codegen

% y = [sqrt(u(1));sqrt(u(2));sqrt(u(3));sqrt(u(4));sqrt(u(5));sqrt(u(6));]/(2*pi);

y = [sqrt(abs(u(1)));sqrt(abs(u(6)));sqrt(abs(u(5)));sqrt(abs(u(4)));sqrt(abs(u(3)));sqrt(abs(u(2)));];

== matlab function hexa_control/Controller1/Controller1 ==
  settings: updateMethod=DISCRETE
  data: f_r output; p input; v input; R input; p_d input; w output; dotp_d input; ddotp_d input; R_r input; u2 output; m parameter; J parameter; g parameter; K_p parameter; K_v parameter; K_R parameter; K_w parameter; e_p output; e_v output; e_R output; e_omega output; feedforward output; feedforward2 output; F parameter
function [f_r,w,u2,e_p,e_v,e_R,e_omega,feedforward,feedforward2] = fcn(p,v,R,p_d,dotp_d,ddotp_d,R_r,m,J,g,K_p,K_v,K_R,K_w, F)


dotp = v(1:3);
omega_B = v(4:6);


e3=[0;0;1];
e_p = p - p_d;
e_v = dotp - dotp_d;
f_r = m*ddotp_d + m*g*e3 - K_p*e_p - K_v*e_v;

omega_d = [0; 0; 0];
dotomega_d = [0; 0; 0];


% rotation error
e_R = 1/2*unskew(R_r.'*R-R.'*R_r); 
e_omega = omega_B - R'*R_r*omega_d;


% feedforward term on omega_d and dotomega_d of the Control
feedforward = - J*(skew(omega_B)*R'*R_r*omega_d - R'*R_r*dotomega_d); %Put in again!!!
feedforward2 = - J*(skew(omega_B)*R'*R_r*omega_d); %Put in again!!!
feedforward=[0 0 0]';


% second output of the Controller (torque)
u2 = cross(omega_B,J*omega_B) - K_R*e_R - K_w*e_omega + feedforward;

% u2  = [-u2(1); u2(2); u2(3)];


w = F^-1 * [R'*f_r; u2];



function res=skew(u)

res=[0 -u(3) u(2);
    u(3) 0 -u(1);
    -u(2) u(1) 0];

function res=unskew(u)

res=[u(3,2);
    u(1,3);
    u(2,1)];
